simulink model "power_system_1"  (R2025b)
settings: Solver=ode23tb  StartTime=0.0  StopTime=0.1  FixedStep=tc  MaxStep=tc
values from neighbouring files (symbols this model uses):
  ts_afe = 1/fPWM_AFE/2    (= 0.000125)    [init_model.m]
undefined symbols (not defined in the file or in its folder): omega_grid_nom
libraries: fl_lib x29, nesl_utility x10, three_windings_transformer x6, dual_threephase_voltage_current_measure x1, three_phase_voltage_emulator x1, power_meter_iec x1
settings Model: SimulationMode=accelerator  Creator=dbagn  LastModifiedBy=dbagn
settings SolverCC: NumberNewtonIterations=3.0  ZeroCrossControl=DisableAll  AlgebraicLoopSolver=TrustRegion  SolverResetMethod=Robust
settings DataIOCC: SaveOutput=off  SignalLogging=off  DSMLogging=off  SaveTime=off  ReturnWorkspaceOutputs=off
settings OptimizationCC: ReuseModelBlockBuffer=off
settings DebuggingCC: UnconnectedInputMsg=warning  UnconnectedOutputMsg=warning  UnconnectedLineMsg=warning
settings ModelReferenceCC: EnableRefExpFcnMdlSchedulingChecks=on
settings SFSimCC: CustomCodeUndefinedFunction=ThrowError  DefaultCustomCodeDeterministicFunctions=All
settings SFSimCC: SimCustomHeaderCode=|
  | #include "rpi.h"
  | #include "mavgflt.h"
  | #include "mavgflt_simulink.h"
  | #include "mavgflts.h"
  | #include "mavgflts_simulink.h"
  | #include "dsmavgflt.h"
  | #include "dsmavgflt_simulink.h"
  | #include "bemf_obsv.h"
  | #include "bemf_obsv_simulink.h"
  | #include "bemf_obsv_load_est.h"
  | #include "bemf_obsv_load_est_simulink.h"
  | #include "dqvector_pi.h"
  | #include "dqvector_pi_simulink.h"
  | #include "sv_pwm_simulink.h"
  | #include "sv_pwm.h"
  | #include "first_harmonic_tracker.h"
  | #include "first_harmonic_tracker_simulink.h"
  | #include "dqpll_thyr.h"
  | #include "dqpll_thyr_simulink.h"
  | #include "dqpll_grid.h"
  | #include "dqpll_grid_simulink.h"
settings SFSimCC: SimUserSources=|
  | "rpi.c"
  | "mavgflt_simulink.c"
  | "mavgflt.c"
  | "mavgflts_simulink.c"
  | "mavgflts.c"
  | "dsmavgflt_simulink.c"
  | "dsmavgflt.c"
  | "bemf_obsv_simulink.c"
  | "bemf_obsv.c"
  | "bemf_obsv_load_est_simulink.c"
  | "bemf_obsv_load_est.c"
  | "dqvector_pi.c"
  | "dqvector_pi_simulink.c"
  | "sv_pwm_simulink.c"
  | "sv_pwm.c"
  | "first_harmonic_tracker_simulink.c"
  | "first_harmonic_tracker.c"
  | "dqpll_thyr_simulink.c"
  | "dqpll_thyr.c"
  | "dqpll_grid_simulink.c"
  | "dqpll_grid.c"
settings SFSimCC: SimUserIncludeDirs=|
  | include
  | src
settings RTWCC: GPUComputeCapability=3.5  DLArmComputeVersion=19.05

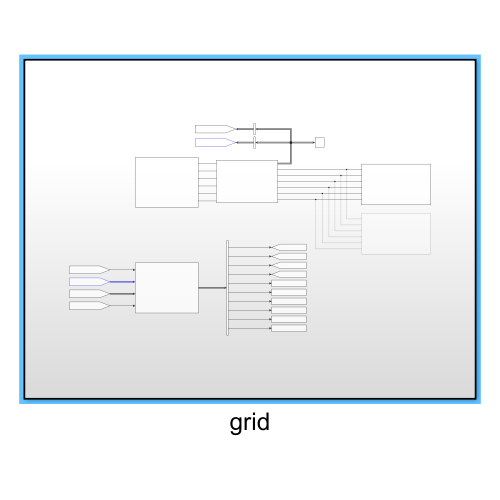
[thumbnail: Simulink's stored preview of the top-level diagram]
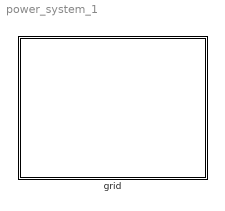
== system power_system_1 ==
  grid : Subsystem

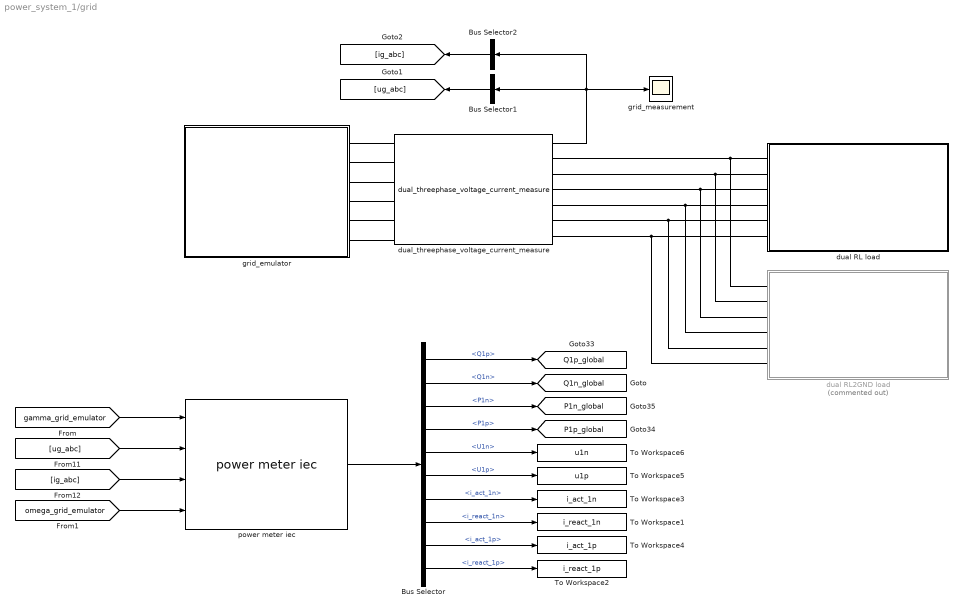
== system power_system_1/grid ==
  Bus Selector : BusSelector  OutputSignals=Q1p,Q1n,P1n,P1p,U1n,U1p,i_act_1n,i_react_1n,i_act_1p,i_react_1p
  Bus Selector1 : BusSelector  OutputSignals=uu12,uv12,uw12  OutputAsBus=on
  Bus Selector2 : BusSelector  OutputSignals=iu,iv,iw  OutputAsBus=on
  To Workspace1 : ToWorkspace  VariableName=i_react_1n  SampleTime=ts_afe
      settings: MaxDataPoints=Ns_afe
  To Workspace2 : ToWorkspace  VariableName=i_react_1p  SampleTime=ts_afe
      settings: MaxDataPoints=Ns_afe
  To Workspace3 : ToWorkspace  VariableName=i_act_1n  SampleTime=ts_afe
      settings: MaxDataPoints=Ns_afe
  To Workspace4 : ToWorkspace  VariableName=i_act_1p  SampleTime=ts_afe
      settings: MaxDataPoints=Ns_afe
  To Workspace5 : ToWorkspace  VariableName=u1p  SampleTime=ts_afe
      settings: MaxDataPoints=Ns_afe
  To Workspace6 : ToWorkspace  VariableName=u1n  SampleTime=ts_afe
      settings: MaxDataPoints=Ns_afe
  dual RL load : Subsystem  mask{Ls_load=1e-3, Rs_load=1}
      mask prompts: Ls_load "Ls_load (H)"; Rs_load "Rs_load (Ohm)"
      mask Display:
      | disp('Dual Three Phase RL Load');
      | port_label('lconn', 1, 'UU1');
      | port_label('lconn', 2, 'UU2');
      | port_label('lconn', 3, 'UV1');
      | port_label('lconn', 4, 'UV2');
      | port_label('lconn', 5, 'UW1');
      | port_label('lconn', 6, 'UW2');
  dual RL2GND load : Subsystem  Commented=on  mask{Ls_load=1e-3, Rs_load=1}
      mask prompts: Ls_load "Ls_load (H)"; Rs_load "Rs_load (Ohm)"
      mask Display:
      | disp('Dual Three Phase RL Load');
      | port_label('lconn', 1, 'UU1');
      | port_label('lconn', 2, 'UU2');
      | port_label('lconn', 3, 'UV1');
      | port_label('lconn', 4, 'UV2');
      | port_label('lconn', 5, 'UW1');
      | port_label('lconn', 6, 'UW2');
  dual_threephase_voltage_current_measure : dual_threephase_voltage_current_measure/dual_threephase_voltage_current_measure
  grid_emulator : Subsystem
  grid_measurement : Scope
      settings: ActiveDisplayYMinimum=-825.55916468412317  ActiveDisplayYMaximum=720.77250310886961
  power meter iec : power_meter_iec/power meter iec  period=pi/omega_grid_nom  ts=ts_afe  enable_time=0.025
  tag scope: P1n_global=global, P1p_global=global, Q1n_global=global, Q1p_global=global
  wires:
  [gamma_grid_emulator] -> power meter iec/1
  [ug_abc] -> power meter iec/2
  [ig_abc] -> power meter iec/3
  power meter iec/1 -> Bus Selector/1
  Bus Selector/1 -> [Q1p_global]  "<Q1p>"
  Bus Selector/2 -> [Q1n_global]  "<Q1n>"
  Bus Selector/3 -> [P1n_global]  "<P1n>"
  Bus Selector/4 -> [P1p_global]  "<P1p>"
  Bus Selector/5 -> To Workspace6/1  "<U1n>"
  Bus Selector/6 -> To Workspace5/1  "<U1p>"
  Bus Selector/7 -> To Workspace3/1  "<i_act_1n>"
  Bus Selector/8 -> To Workspace1/1  "<i_react_1n>"
  Bus Selector/9 -> To Workspace4/1  "<i_act_1p>"
  Bus Selector/10 -> To Workspace2/1  "<i_react_1p>"
  [omega_grid_emulator] -> power meter iec/4
  dual_threephase_voltage_current_measure/1 -> grid_measurement/1, Bus Selector1/1, Bus Selector2/1
  Bus Selector1/1 -> [ug_abc]
  Bus Selector2/1 -> [ig_abc]
  connections:
  dual_threephase_voltage_current_measure/LConn6 -- grid_emulator/RConn6
  dual_threephase_voltage_current_measure/LConn5 -- grid_emulator/RConn5
  dual_threephase_voltage_current_measure/LConn4 -- grid_emulator/RConn4
  dual_threephase_voltage_current_measure/LConn3 -- grid_emulator/RConn3
  dual_threephase_voltage_current_measure/LConn2 -- grid_emulator/RConn2
  dual_threephase_voltage_current_measure/LConn1 -- grid_emulator/RConn1
  dual RL load/LConn1 -- dual RL2GND load/LConn1 -- dual_threephase_voltage_current_measure/RConn1
  dual RL load/LConn2 -- dual RL2GND load/LConn2 -- dual_threephase_voltage_current_measure/RConn2
  dual RL load/LConn3 -- dual RL2GND load/LConn3 -- dual_threephase_voltage_current_measure/RConn3
  dual RL load/LConn4 -- dual RL2GND load/LConn4 -- dual_threephase_voltage_current_measure/RConn4
  dual RL load/LConn5 -- dual RL2GND load/LConn5 -- dual_threephase_voltage_current_measure/RConn5
  dual RL load/LConn6 -- dual RL2GND load/LConn6 -- dual_threephase_voltage_current_measure/RConn6

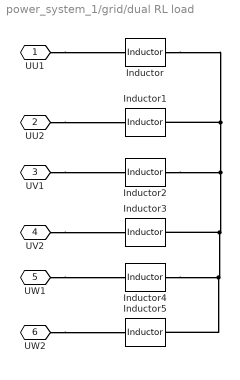
== system power_system_1/grid/dual RL load ==
  Inductor{,1..5} (6 alike) : fl_lib/Electrical/Electrical Elements/Inductor  l=Ls_load H  r=Rs_load Ohm  g=1e-9 1/Ohm  i_specify=off  i_priority=None  i=0 A  i_nominal_specify=off  i_nominal_value=1  i_nominal_unit=A  v_specify=off  v_priority=None  v=0 V  v_nominal_specify=off  v_nominal_value=1  v_nominal_unit=V  i_L_specify=off  i_L_priority=High  i_L=0 A  i_L_nominal_specify=off  i_L_nominal_value=1  i_L_nominal_unit=A
  UU1 : PMIOPort  Side=Left
  UU2 : PMIOPort  Port=2  Side=Left
  UV1 : PMIOPort  Port=3  Side=Left
  UV2 : PMIOPort  Port=4  Side=Left
  UW1 : PMIOPort  Port=5  Side=Left
  UW2 : PMIOPort  Port=6  Side=Left
  connections:
  Inductor/RConn1 -- Inductor4/RConn1 -- Inductor5/RConn1 -- Inductor3/RConn1 -- Inductor2/RConn1 -- Inductor1/RConn1
  UV2/RConn1 -- Inductor3/LConn1
  UU1/RConn1 -- Inductor/LConn1
  UW2/RConn1 -- Inductor5/LConn1
  UU2/RConn1 -- Inductor1/LConn1
  UW1/RConn1 -- Inductor4/LConn1
  UV1/RConn1 -- Inductor2/LConn1

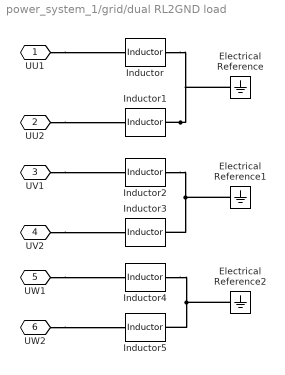
== system power_system_1/grid/dual RL2GND load ==
  Electrical Reference : fl_lib/Electrical/Electrical Elements/Electrical Reference
  Electrical Reference1 : fl_lib/Electrical/Electrical Elements/Electrical Reference
  Electrical Reference2 : fl_lib/Electrical/Electrical Elements/Electrical Reference
  Inductor{,1..5} (6 alike) : fl_lib/Electrical/Electrical Elements/Inductor  l=Ls_load H  r=Rs_load Ohm  g=1e-9 1/Ohm  i_specify=off  i_priority=None  i=0 A  i_nominal_specify=off  i_nominal_value=1  i_nominal_unit=A  v_specify=off  v_priority=None  v=0 V  v_nominal_specify=off  v_nominal_value=1  v_nominal_unit=V  i_L_specify=off  i_L_priority=High  i_L=0 A  i_L_nominal_specify=off  i_L_nominal_value=1  i_L_nominal_unit=A
  UU1 : PMIOPort  Side=Left
  UU2 : PMIOPort  Port=2  Side=Left
  UV1 : PMIOPort  Port=3  Side=Left
  UV2 : PMIOPort  Port=4  Side=Left
  UW1 : PMIOPort  Port=5  Side=Left
  UW2 : PMIOPort  Port=6  Side=Left
  connections:
  UV1/RConn1 -- Inductor2/LConn1
  UW1/RConn1 -- Inductor4/LConn1
  UU2/RConn1 -- Inductor1/LConn1
  UW2/RConn1 -- Inductor5/LConn1
  UU1/RConn1 -- Inductor/LConn1
  Inductor1/RConn1 -- Electrical Reference/LConn1 -- Inductor/RConn1
  UV2/RConn1 -- Inductor3/LConn1
  Electrical Reference2/LConn1 -- Inductor5/RConn1 -- Inductor4/RConn1
  Electrical Reference1/LConn1 -- Inductor3/RConn1 -- Inductor2/RConn1

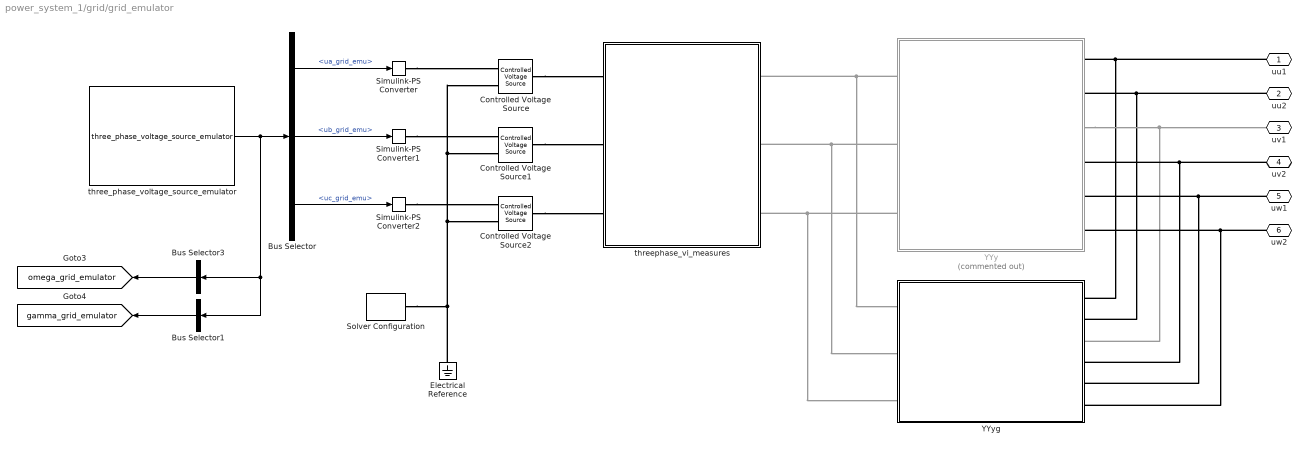
== system power_system_1/grid/grid_emulator ==
  Bus Selector : BusSelector  OutputSignals=ua_grid_emu,ub_grid_emu,uc_grid_emu
  Bus Selector1 : BusSelector  OutputSignals=gamma_grid_emulator  OutputAsBus=on
  Bus Selector3 : BusSelector  OutputSignals=omega_grid_emulator  OutputAsBus=on
  Controlled Voltage Source : fl_lib/Electrical/Electrical Sources/Controlled Voltage Source
  Controlled Voltage Source1 : fl_lib/Electrical/Electrical Sources/Controlled Voltage Source
  Controlled Voltage Source2 : fl_lib/Electrical/Electrical Sources/Controlled Voltage Source
  Electrical Reference : fl_lib/Electrical/Electrical Elements/Electrical Reference
  Simulink-PS Converter : nesl_utility/Simulink-PS Converter  PhysicalDomain=network_engine_domain  SubClassName=ps_input  LeftPortType=input  RightPortType=output  PseudoPeriodic=off  Frequencies=[]  NoiseDistribution=none  NoiseParameters=[]  Unit=V  AffineConversion=on  FilteringAndDerivatives=provide  SimscapeFilterOrder=1  InputFilterTimeConstant=0.001  UdotUserProvided=0
  Simulink-PS Converter1 : nesl_utility/Simulink-PS Converter  PhysicalDomain=network_engine_domain  SubClassName=ps_input  LeftPortType=input  RightPortType=output  PseudoPeriodic=off  Frequencies=[]  NoiseDistribution=none  NoiseParameters=[]  Unit=V  AffineConversion=on  FilteringAndDerivatives=provide  SimscapeFilterOrder=1  InputFilterTimeConstant=0.001  UdotUserProvided=0
  Simulink-PS Converter2 : nesl_utility/Simulink-PS Converter  PhysicalDomain=network_engine_domain  SubClassName=ps_input  LeftPortType=input  RightPortType=output  PseudoPeriodic=off  Frequencies=[]  NoiseDistribution=none  NoiseParameters=[]  Unit=V  AffineConversion=on  FilteringAndDerivatives=provide  SimscapeFilterOrder=1  InputFilterTimeConstant=0.001  UdotUserProvided=0
  Solver Configuration : nesl_utility/Solver Configuration  PhysicalDomain=network_engine_domain  SubClassName=solver  LeftPortType=input  RightPortType=generic  Tones=[]  Harmonics=[]  SimulateNoise=off  Profile=off  UseLocalSampling=off  EnableSwitchedLinearOptims=on  FrequencyDomain=off  UseCCode=off  RelTol=0.001  AbsTol=0.001  MinStep=1e-09  ToWorkspace=off  RevertToSquareIcSolve=off  NumHomotopyIterations=100  PhasorMode=off  PhasorModeNumHarmonics=1  ConsistencySolver=NEWTON_FTOL  IndexReductionMethod=DerivativeReplacement  DoDC=on  ResidualTolerance=1e-3  ConsistencyTolSource=GLOBAL  ConsistencyAbsTol=0.001  ConsistencyRelTol=0.001  ConsistencyTolFactor=0.001  UseLocalSolver=on  LocalSolverChoice=NE_BACKWARD_EULER_ADVANCER  ResolveIndetEquations=on  FunctionEvalNumThread=1  LocalSolverSampleTime=tc  DoFixedCost=on  MaxNonlinIter=3  MaxModeIter=2  ComputeImpulses=off  ImpulseIterations=2  LinearAlgebra=auto  LinearAlgebraNumThread=0  EquationFormulation=NE_TIME_EF  DelaysMemoryBudget=1024  AutomaticFiltering=on  FilteringTimeConstant=0.001  PartitionStorageMethod=AS_NEEDED  PartitionMemoryBudget=1024  PartitionMethod=ROBUST  MultibodyUseLocalSolver=off  MultibodyLocalSolverChoice=ODE1  MultibodyLocalSolverSampleTime=0.001
  YYy : Subsystem  Commented=on
  YYyg : Subsystem
  three_phase_voltage_source_emulator : three_phase_voltage_emulator/three_phase_voltage_source_emulator  freq=50  ugrid_nom=690  vp_xi_pu=1  vp_eta_pu=0  vn_xi_pu=0  vn_eta_pu=0  fcut_lvrt=50
  threephase_vi_measures : Subsystem
  uu1 : PMIOPort  Side=Right
  uu2 : PMIOPort  Port=2  Side=Right
  uv1 : PMIOPort  Port=3  Side=Right
  uv2 : PMIOPort  Port=4  Side=Right
  uw1 : PMIOPort  Port=5  Side=Right
  uw2 : PMIOPort  Port=6  Side=Right
  tag scope: gamma_grid_emulator=global, omega_grid_emulator=global
  wires:
  Bus Selector/2 -> Simulink-PS Converter1/1  "<ub_grid_emu>"
  Bus Selector/3 -> Simulink-PS Converter2/1  "<uc_grid_emu>"
  Bus Selector/1 -> Simulink-PS Converter/1  "<ua_grid_emu>"
  three_phase_voltage_source_emulator/1 -> Bus Selector1/1, Bus Selector3/1, Bus Selector/1
  Bus Selector3/1 -> [omega_grid_emulator]
  Bus Selector1/1 -> [gamma_grid_emulator]
  connections:
  Simulink-PS Converter/RConn1 -- Controlled Voltage Source/RConn1
  Simulink-PS Converter1/RConn1 -- Controlled Voltage Source1/RConn1
  Simulink-PS Converter2/RConn1 -- Controlled Voltage Source2/RConn1
  Electrical Reference/LConn1 -- Controlled Voltage Source/RConn2 -- Controlled Voltage Source1/RConn2 -- Controlled Voltage Source2/RConn2 -- Solver Configuration/RConn1
  YYy/LConn1 -- YYyg/LConn1 -- threephase_vi_measures/RConn1
  YYy/LConn2 -- YYyg/LConn2 -- threephase_vi_measures/RConn2
  YYy/LConn3 -- YYyg/LConn3 -- threephase_vi_measures/RConn3
  Controlled Voltage Source/LConn1 -- threephase_vi_measures/LConn1
  Controlled Voltage Source1/LConn1 -- threephase_vi_measures/LConn2
  Controlled Voltage Source2/LConn1 -- threephase_vi_measures/LConn3
  uu1/RConn1 -- YYyg/RConn1 -- YYy/RConn1
  uu2/RConn1 -- YYyg/RConn2 -- YYy/RConn2
  YYy/RConn3 -- YYyg/RConn3 -- uv1/RConn1
  uv2/RConn1 -- YYyg/RConn4 -- YYy/RConn4
  uw1/RConn1 -- YYyg/RConn5 -- YYy/RConn5
  uw2/RConn1 -- YYyg/RConn6 -- YYy/RConn6

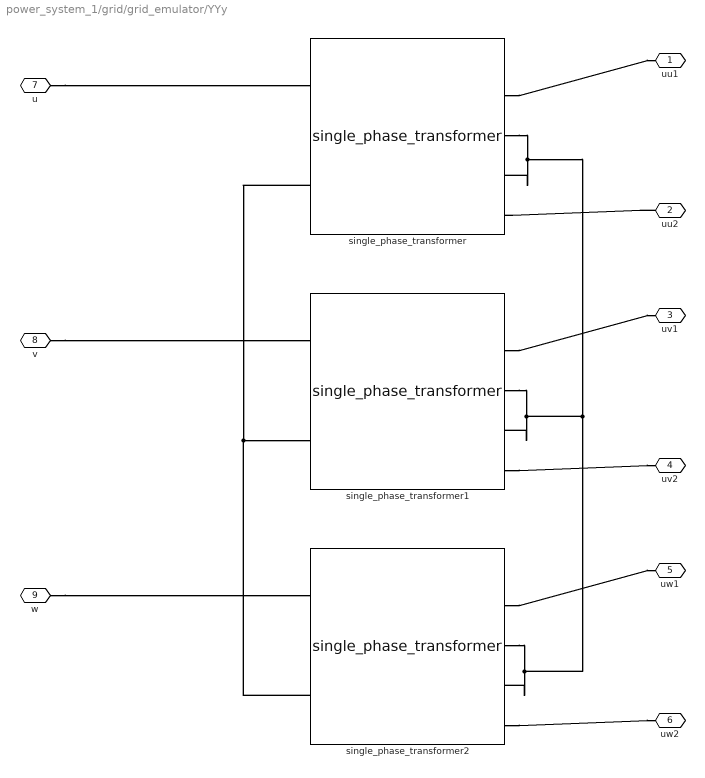
== system power_system_1/grid/grid_emulator/YYy ==
  single_phase_transformer : three_windings_transformer/single_phase_transformer  lm_trafo=1e-3  m1=6  m2=3  m3=3  rd1_trafo=1e-3  rd2_trafo=1e-3  rd3_trafo=1e-3  ld1_trafo=6e-6  ld2_trafo=12e-6  ld3_trafo=12e-6  rfe_trafo=1e3  length_core=0.5  mu0=1.256637e-6  mur=70
  single_phase_transformer1 : three_windings_transformer/single_phase_transformer  lm_trafo=1e-3  m1=6  m2=3  m3=3  rd1_trafo=1e-3  rd2_trafo=1e-3  rd3_trafo=1e-3  ld1_trafo=6e-6  ld2_trafo=12e-6  ld3_trafo=12e-6  rfe_trafo=1e3  length_core=0.5  mu0=1.256637e-6  mur=70
  single_phase_transformer2 : three_windings_transformer/single_phase_transformer  lm_trafo=1e-3  m1=6  m2=3  m3=3  rd1_trafo=1e-3  rd2_trafo=1e-3  rd3_trafo=1e-3  ld1_trafo=6e-6  ld2_trafo=12e-6  ld3_trafo=12e-6  rfe_trafo=1e3  length_core=0.5  mu0=1.256637e-6  mur=70
  uu1 : PMIOPort  Side=Right
  uu2 : PMIOPort  Port=2  Side=Right
  uv1 : PMIOPort  Port=3  Side=Right
  uv2 : PMIOPort  Port=4  Side=Right
  uw1 : PMIOPort  Port=5  Side=Right
  uw2 : PMIOPort  Port=6  Side=Right
  u : PMIOPort  Port=7  Side=Left
  v : PMIOPort  Port=8  Side=Left
  w : PMIOPort  Port=9  Side=Left
  connections:
  single_phase_transformer1/RConn4 -- uv2/RConn1
  single_phase_transformer1/RConn1 -- uv1/RConn1
  single_phase_transformer/RConn1 -- uu1/RConn1
  uu2/RConn1 -- single_phase_transformer/RConn4
  single_phase_transformer2/RConn4 -- uw2/RConn1
  single_phase_transformer/RConn2 -- single_phase_transformer/RConn3 -- single_phase_transformer2/RConn3 -- single_phase_transformer2/RConn2 -- single_phase_transformer1/RConn2 -- single_phase_transformer1/RConn3
  single_phase_transformer2/RConn1 -- uw1/RConn1
  u/RConn1 -- single_phase_transformer/LConn1
  v/RConn1 -- single_phase_transformer1/LConn1
  w/RConn1 -- single_phase_transformer2/LConn1
  single_phase_transformer/LConn2 -- single_phase_transformer1/LConn2 -- single_phase_transformer2/LConn2

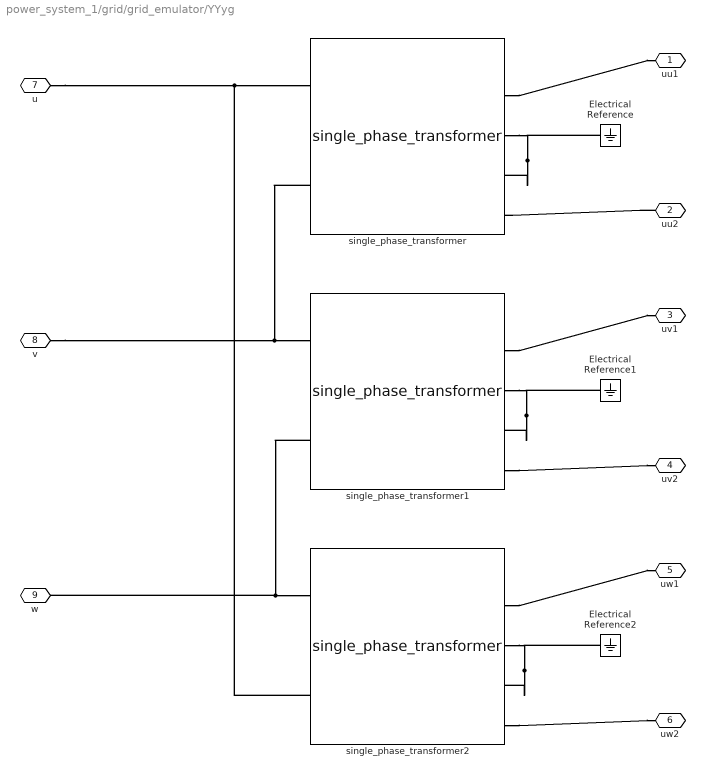
== system power_system_1/grid/grid_emulator/YYyg ==
  Electrical Reference : fl_lib/Electrical/Electrical Elements/Electrical Reference
  Electrical Reference1 : fl_lib/Electrical/Electrical Elements/Electrical Reference
  Electrical Reference2 : fl_lib/Electrical/Electrical Elements/Electrical Reference
  single_phase_transformer : three_windings_transformer/single_phase_transformer  lm_trafo=1e-3  m1=6  m2=3  m3=3  rd1_trafo=1e-3  rd2_trafo=1e-3  rd3_trafo=1e-3  ld1_trafo=6e-6  ld2_trafo=12e-6  ld3_trafo=12e-6  rfe_trafo=1e3  length_core=0.5  mu0=1.256637e-6  mur=70
  single_phase_transformer1 : three_windings_transformer/single_phase_transformer  lm_trafo=1e-3  m1=6  m2=3  m3=3  rd1_trafo=1e-3  rd2_trafo=1e-3  rd3_trafo=1e-3  ld1_trafo=6e-6  ld2_trafo=12e-6  ld3_trafo=12e-6  rfe_trafo=1e3  length_core=0.5  mu0=1.256637e-6  mur=70
  single_phase_transformer2 : three_windings_transformer/single_phase_transformer  lm_trafo=1e-3  m1=6  m2=3  m3=3  rd1_trafo=1e-3  rd2_trafo=1e-3  rd3_trafo=1e-3  ld1_trafo=6e-6  ld2_trafo=12e-6  ld3_trafo=12e-6  rfe_trafo=1e3  length_core=0.5  mu0=1.256637e-6  mur=70
  uu1 : PMIOPort  Side=Right
  uu2 : PMIOPort  Port=2  Side=Right
  uv1 : PMIOPort  Port=3  Side=Right
  uv2 : PMIOPort  Port=4  Side=Right
  uw1 : PMIOPort  Port=5  Side=Right
  uw2 : PMIOPort  Port=6  Side=Right
  u : PMIOPort  Port=7  Side=Left
  v : PMIOPort  Port=8  Side=Left
  w : PMIOPort  Port=9  Side=Left
  connections:
  u/RConn1 -- single_phase_transformer2/LConn2 -- single_phase_transformer/LConn1
  single_phase_transformer1/RConn2 -- Electrical Reference1/LConn1 -- single_phase_transformer1/RConn3
  single_phase_transformer2/RConn1 -- uw1/RConn1
  single_phase_transformer/RConn2 -- Electrical Reference/LConn1 -- single_phase_transformer/RConn3
  single_phase_transformer2/RConn2 -- Electrical Reference2/LConn1 -- single_phase_transformer2/RConn3
  single_phase_transformer2/RConn4 -- uw2/RConn1
  uu2/RConn1 -- single_phase_transformer/RConn4
  single_phase_transformer/RConn1 -- uu1/RConn1
  single_phase_transformer1/RConn1 -- uv1/RConn1
  single_phase_transformer1/RConn4 -- uv2/RConn1
  single_phase_transformer/LConn2 -- single_phase_transformer1/LConn1 -- v/RConn1
  single_phase_transformer1/LConn2 -- single_phase_transformer2/LConn1 -- w/RConn1

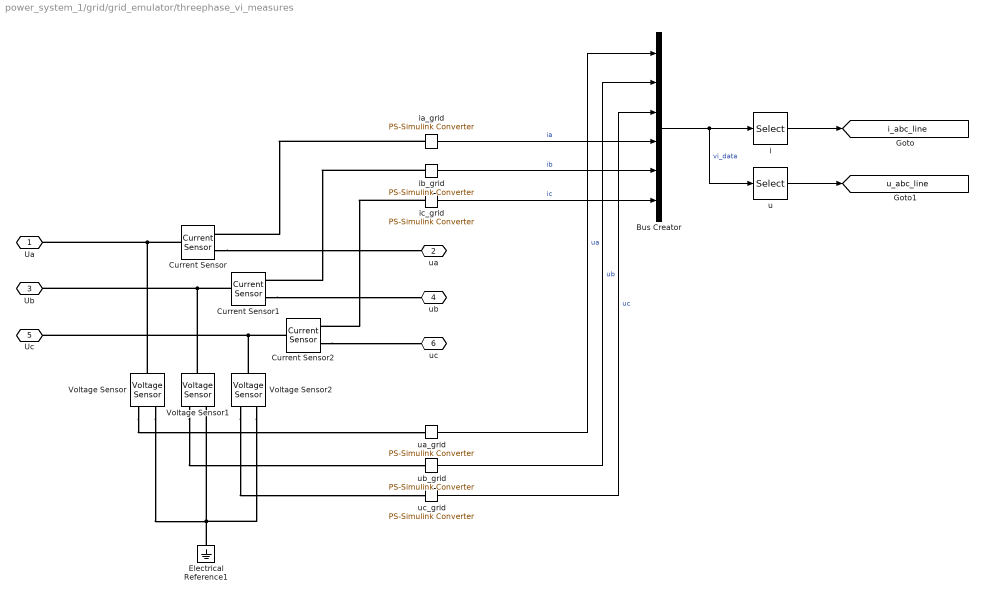
== system power_system_1/grid/grid_emulator/threephase_vi_measures ==
  Bus Creator : BusCreator  Inputs=6
  Current Sensor : fl_lib/Electrical/Electrical Sensors/Current Sensor
  Current Sensor1 : fl_lib/Electrical/Electrical Sensors/Current Sensor
  Current Sensor2 : fl_lib/Electrical/Electrical Sensors/Current Sensor
  Electrical Reference1 : fl_lib/Electrical/Electrical Elements/Electrical Reference
  Voltage Sensor : fl_lib/Electrical/Electrical Sensors/Voltage Sensor
  Voltage Sensor1 : fl_lib/Electrical/Electrical Sensors/Voltage Sensor
  Voltage Sensor2 : fl_lib/Electrical/Electrical Sensors/Voltage Sensor
  i : Selector  InputPortWidth=6  IndexOptions=Index vector (dialog)  Indices=[4 5 6]  OutputSizes=1
  ia_grid : nesl_utility/PS-Simulink Converter  PhysicalDomain=network_engine_domain  SubClassName=ps_output  LeftPortType=input  RightPortType=output  PseudoPeriodic=off  Frequencies=[]  VectorFormat=1-D array  Unit=A  AffineConversion=off
  ib_grid : nesl_utility/PS-Simulink Converter  PhysicalDomain=network_engine_domain  SubClassName=ps_output  LeftPortType=input  RightPortType=output  PseudoPeriodic=off  Frequencies=[]  VectorFormat=1-D array  Unit=A  AffineConversion=off
  ic_grid : nesl_utility/PS-Simulink Converter  PhysicalDomain=network_engine_domain  SubClassName=ps_output  LeftPortType=input  RightPortType=output  PseudoPeriodic=off  Frequencies=[]  VectorFormat=1-D array  Unit=A  AffineConversion=off
  u : Selector  InputPortWidth=6  IndexOptions=Index vector (dialog)  Indices=[1 2 3]  OutputSizes=1
  ua_grid : nesl_utility/PS-Simulink Converter  PhysicalDomain=network_engine_domain  SubClassName=ps_output  LeftPortType=input  RightPortType=output  PseudoPeriodic=off  Frequencies=[]  VectorFormat=1-D array  Unit=V  AffineConversion=off
  ub_grid : nesl_utility/PS-Simulink Converter  PhysicalDomain=network_engine_domain  SubClassName=ps_output  LeftPortType=input  RightPortType=output  PseudoPeriodic=off  Frequencies=[]  VectorFormat=1-D array  Unit=V  AffineConversion=off
  uc_grid : nesl_utility/PS-Simulink Converter  PhysicalDomain=network_engine_domain  SubClassName=ps_output  LeftPortType=input  RightPortType=output  PseudoPeriodic=off  Frequencies=[]  VectorFormat=1-D array  Unit=V  AffineConversion=off
  Ua : PMIOPort  Side=Left
  ua : PMIOPort  Port=2  Side=Right
  Ub : PMIOPort  Port=3  Side=Left
  ub : PMIOPort  Port=4  Side=Right
  Uc : PMIOPort  Port=5  Side=Left
  uc : PMIOPort  Port=6  Side=Right
  tag scope: i_abc_line=global, u_abc_line=global
  wires:
  Bus Creator/1 -> i/1, u/1  "vi_data"
  ib_grid/1 -> Bus Creator/5  "ib"
  ia_grid/1 -> Bus Creator/4  "ia"
  ic_grid/1 -> Bus Creator/6  "ic"
  ua_grid/1 -> Bus Creator/1  "ua"
  ub_grid/1 -> Bus Creator/2  "ub"
  uc_grid/1 -> Bus Creator/3  "uc"
  i/1 -> [i_abc_line]
  u/1 -> [u_abc_line]
  connections:
  Current Sensor1/LConn1 -- Ub/RConn1 -- Voltage Sensor1/LConn1
  Electrical Reference1/LConn1 -- Voltage Sensor/RConn2 -- Voltage Sensor2/RConn2 -- Voltage Sensor1/RConn2
  Voltage Sensor/RConn1 -- ua_grid/LConn1
  Current Sensor/RConn2 -- ua/RConn1
  Voltage Sensor1/RConn1 -- ub_grid/LConn1
  Voltage Sensor2/LConn1 -- Current Sensor2/LConn1 -- Uc/RConn1
  Current Sensor/LConn1 -- Ua/RConn1 -- Voltage Sensor/LConn1
  Current Sensor1/RConn2 -- ub/RConn1
  Voltage Sensor2/RConn1 -- uc_grid/LConn1
  ib_grid/LConn1 -- Current Sensor1/RConn1
  ia_grid/LConn1 -- Current Sensor/RConn1
  ic_grid/LConn1 -- Current Sensor2/RConn1
  Current Sensor2/RConn2 -- uc/RConn1
